simulink model "linearTFSimplifiedDecoupling"  (Simulink 7.7)
settings: Solver=ode45  StartTime=0.0  StopTime=700  RelTol=1e-3
values from neighbouring files (symbols this model uses):
  QT =     [FaseMinima.mat]    (also in FaseNaoMinima.mat; FaseNaoMinimaMudandoApenasGama.mat; settup.m = dynamics())
libraries: simulink x2
settings Model: Creator=Arthur  LastModifiedBy=Arthur

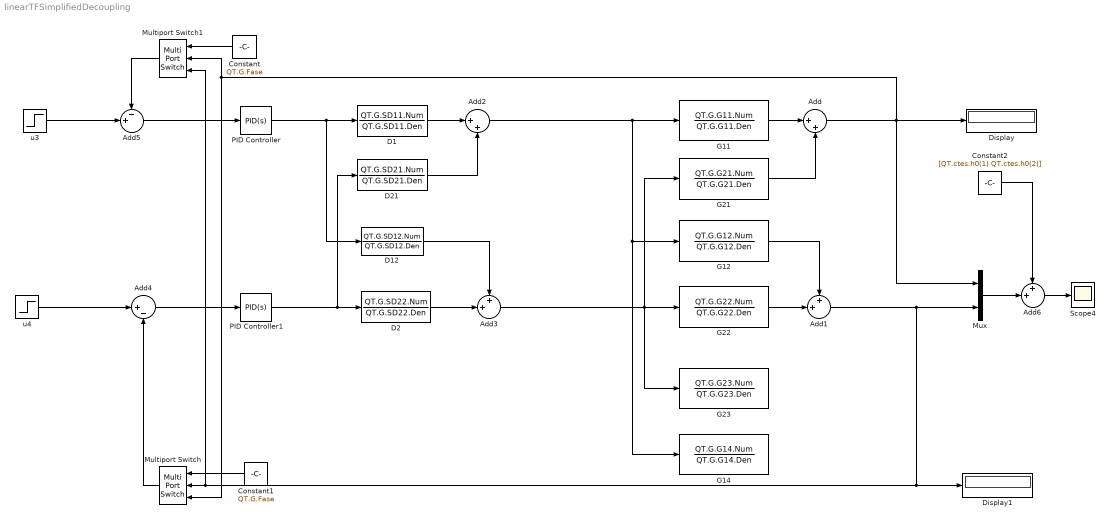
== system linearTFSimplifiedDecoupling ==
  Add : Sum  Inputs=|++
  Add1 : Sum  Inputs=++|
  Add2 : Sum  Inputs=|++
  Add3 : Sum  Inputs=++|
  Add4 : Sum  Inputs=|+-
  Add5 : Sum  Inputs=-+|
  Add6 : Sum  Inputs=++|
  Constant : Constant  Value=QT.G.Fase
  Constant1 : Constant  Value=QT.G.Fase
  Constant2 : Constant  Value=[QT.ctes.h0(1) QT.ctes.h0(2)]
  D1 : TransferFcn  Numerator=QT.G.SD11.Num  Denominator=QT.G.SD11.Den
  D12 : TransferFcn  Numerator=QT.G.SD12.Num  Denominator=QT.G.SD12.Den
  D2 : TransferFcn  Numerator=QT.G.SD22.Num  Denominator=QT.G.SD22.Den
  D21 : TransferFcn  Numerator=QT.G.SD21.Num  Denominator=QT.G.SD21.Den
  Display : Display
  Display1 : Display
  G11 : TransferFcn  Numerator=QT.G.G11.Num  Denominator=QT.G.G11.Den
  G12 : TransferFcn  Numerator=QT.G.G12.Num  Denominator=QT.G.G12.Den
  G14 : TransferFcn  Numerator=QT.G.G14.Num  Denominator=QT.G.G14.Den
  G21 : TransferFcn  Numerator=QT.G.G21.Num  Denominator=QT.G.G21.Den
  G22 : TransferFcn  Numerator=QT.G.G22.Num  Denominator=QT.G.G22.Den
  G23 : TransferFcn  Numerator=QT.G.G23.Num  Denominator=QT.G.G23.Den
  Multiport Switch : MultiPortSwitch  Inputs=2  zeroidx=off
  Multiport Switch1 : MultiPortSwitch  Inputs=2  zeroidx=off
  Mux : Mux  Inputs=2
  PID Controller : simulink/Continuous/PID Controller  SystemSampleTime=-1  Controller=PID  TimeDomain=Continuous-time  SampleTime=1  IntegratorMethod=Forward Euler  FilterMethod=Forward Euler  Form=Parallel  P=QT.G.SDPID1.kp  I=QT.G.SDPID1.ki  D=QT.G.SDPID1.kd  N=100  InitialConditionSource=internal  InitialConditionForIntegrator=0  InitialConditionForFilter=0  ExternalReset=none  LimitOutput=off  UpperSaturationLimit=inf  LowerSaturationLimit=-inf  LinearizeAsGain=off  AntiWindupMode=none  Kb=1  TrackingMode=off  Kt=1  PParamMin=[]  PParamMax=[]  IParamMin=[]  IParamMax=[]  DParamMin=[]  DParamMax=[]  NParamMin=[]  NParamMax=[]  KbParamMin=[]  KbParamMax=[]  KtParamMin=[]  KtParamMax=[]  POutMin=[]  POutMax=[]  IOutMin=[]  IOutMax=[]  DOutMin=[]  DOutMax=[]  NOutMin=[]  NOutMax=[]  KbOutMin=[]  KbOutMax=[]  KtOutMin=[]  KtOutMax=[]  IntegratorOutMin=[]  IntegratorOutMax=[]  FilterOutMin=[]  FilterOutMax=[]  SumOutMin=[]  SumOutMax=[]  SumI1OutMin=[]  SumI1OutMax=[]  SumI2OutMin=[]  SumI2OutMax=[]  SumI3OutMin=[]  SumI3OutMax=[]  SumDOutMin=[]  SumDOutMax=[]  SaturationOutMin=[]  SaturationOutMax=[]  IntegratorContinuousStateAttributes=''  IntegratorStateMustResolveToSignalObject=off  IntegratorRTWStateStorageClass=Auto  FilterContinuousStateAttributes=''  FilterStateMustResolveToSignalObject=off  FilterRTWStateStorageClass=Auto
  PID Controller1 : simulink/Continuous/PID Controller  SystemSampleTime=-1  Controller=PID  TimeDomain=Continuous-time  SampleTime=1  IntegratorMethod=Forward Euler  FilterMethod=Forward Euler  Form=Parallel  P=QT.G.SDPID2.kp  I=QT.G.SDPID2.ki  D=QT.G.SDPID2.kd  N=100  InitialConditionSource=internal  InitialConditionForIntegrator=0  InitialConditionForFilter=0  ExternalReset=none  LimitOutput=off  UpperSaturationLimit=inf  LowerSaturationLimit=-inf  LinearizeAsGain=off  AntiWindupMode=none  Kb=1  TrackingMode=off  Kt=1  PParamMin=[]  PParamMax=[]  IParamMin=[]  IParamMax=[]  DParamMin=[]  DParamMax=[]  NParamMin=[]  NParamMax=[]  KbParamMin=[]  KbParamMax=[]  KtParamMin=[]  KtParamMax=[]  POutMin=[]  POutMax=[]  IOutMin=[]  IOutMax=[]  DOutMin=[]  DOutMax=[]  NOutMin=[]  NOutMax=[]  KbOutMin=[]  KbOutMax=[]  KtOutMin=[]  KtOutMax=[]  IntegratorOutMin=[]  IntegratorOutMax=[]  FilterOutMin=[]  FilterOutMax=[]  SumOutMin=[]  SumOutMax=[]  SumI1OutMin=[]  SumI1OutMax=[]  SumI2OutMin=[]  SumI2OutMax=[]  SumI3OutMin=[]  SumI3OutMax=[]  SumDOutMin=[]  SumDOutMax=[]  SaturationOutMin=[]  SaturationOutMax=[]  IntegratorContinuousStateAttributes=''  IntegratorStateMustResolveToSignalObject=off  IntegratorRTWStateStorageClass=Auto  FilterContinuousStateAttributes=''  FilterStateMustResolveToSignalObject=off  FilterRTWStateStorageClass=Auto
  Scope4 : Scope
      settings: TimeRange=10  SaveName=Simulado
  u3 : Step  Time=200  SampleTime=0
  u4 : Step  Time=500  SampleTime=0
  wires:
  G11/1 -> Add/1
  G21/1 -> Add/2
  G22/1 -> Add1/2
  G12/1 -> Add1/1
  Add/1 -> Display/1, Multiport Switch/3, Multiport Switch1/2, Mux/1
  Add2/1 -> G11/1, G12/1, G14/1
  D21/1 -> Add2/2
  Add1/1 -> Mux/2, Multiport Switch/2, Multiport Switch1/3, Display1/1
  D12/1 -> Add3/1
  Add3/1 -> G22/1, G21/1, G23/1
  Add4/1 -> PID Controller1/1
  Add5/1 -> PID Controller/1
  D1/1 -> Add2/1
  D2/1 -> Add3/2
  Constant/1 -> Multiport Switch1/1
  Constant1/1 -> Multiport Switch/1
  PID Controller/1 -> D12/1, D1/1
  PID Controller1/1 -> D21/1, D2/1
  Multiport Switch/1 -> Add4/2
  Multiport Switch1/1 -> Add5/1
  u3/1 -> Add5/2
  u4/1 -> Add4/1
  Mux/1 -> Add6/2
  Add6/1 -> Scope4/1
  Constant2/1 -> Add6/1
